simulink model "s0401_DC_motor_Torque_Feedback"  (R2021a)
settings: Solver=VariableStepAuto  StartTime=0.0  StopTime=0.2  RelTol=1e-3
libraries: pid_lib x1
settings Model: Creator=s329046  LastModifiedBy=s329046

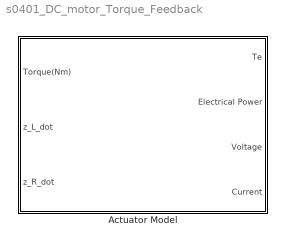
== system s0401_DC_motor_Torque_Feedback ==
  "Actuator Model " : Subsystem

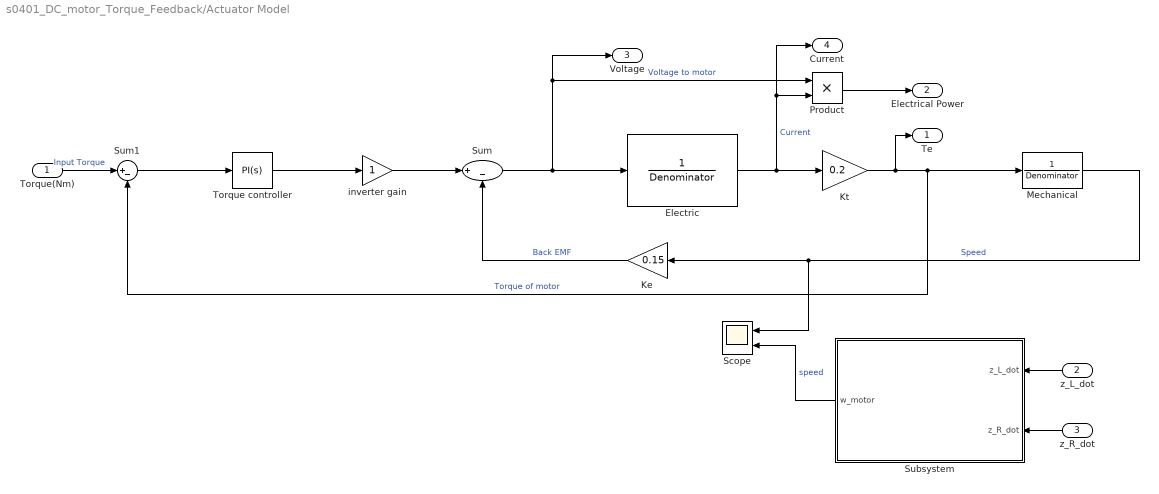
== system s0401_DC_motor_Torque_Feedback/Actuator Model  ==
  Torque(Nm) : Inport
  z_L_dot : Inport  Port=2
  z_R_dot : Inport  Port=3
  "Electric " : TransferFcn  Denominator=Denominator  mask{Denominator=[0.0001 0.8]}
      mask prompts: Denominator "[La Ra]"
      mask TypeOptions Denominator: Denominator
  Ke : Gain  Gain=0.15
  Kt : Gain  Gain=0.2
  Mechanical : TransferFcn  Denominator=Denominator  mask{Denominator=[0.0002 0.042]}
      mask prompts: Denominator "[J B]"
      mask TypeOptions Denominator: Denominator
  Product : Product
  Scope : Scope  NumInputPorts=2
  Subsystem : Subsystem
  Sum : Sum  Inputs=|+-
  Sum1 : Sum  Inputs=|+-
  "Torque controller " : pid_lib/PID Controller  Controller=PI  Form=Parallel  TimeDomain=Continuous-time  UseExternalTs=off  SampleTime=-1  IntegratorMethod=Forward Euler  FilterMethod=Forward Euler  ControllerParametersSource=internal  P=0.59  I=3492  D=0  UseFilter=on  N=100  TunerSelectOption=Transfer Function Based (PID Tuner App)  InitialConditionSource=internal  InitialConditionForIntegrator=0  InitialConditionForFilter=0  DifferentiatorICPrevScaledInput=0  ExternalReset=none  TrackingMode=off  Kt=1  LimitOutput=off  SatLimitsSource=internal  UpperSaturationLimit=inf  LowerSaturationLimit=-inf  LinearizeAsGain=on  AntiWindupMode=none  Kb=1  POutMin=[]  POutMax=[]  IOutMin=[]  IOutMax=[]  DOutMin=[]  DOutMax=[]  NOutMin=[]  NOutMax=[]  SumOutMin=[]  SumOutMax=[]  SaturationOutMin=[]  SaturationOutMax=[]  PParamMin=[]  PParamMax=[]  IParamMin=[]  IParamMax=[]  DParamMin=[]  DParamMax=[]  NParamMin=[]  NParamMax=[]  KbParamMin=[]  KbParamMax=[]  KtParamMin=[]  KtParamMax=[]  KbOutMin=[]  KbOutMax=[]  KtOutMin=[]  KtOutMax=[]  IntegratorOutMin=[]  IntegratorOutMax=[]  FilterOutMin=[]  FilterOutMax=[]  SumI1OutMin=[]  SumI1OutMax=[]  SumI2OutMin=[]  SumI2OutMax=[]  SumI3OutMin=[]  SumI3OutMax=[]  SumI4OutMin=[]  SumI4OutMax=[]  SumDOutMin=[]  SumDOutMax=[]  DifferentiatorOutMin=[]  DifferentiatorOutMax=[]  FilterDiffOutCoefMin=[]  FilterDiffOutCoefMax=[]  ReciprocalOutMin=[]  ReciprocalOutMax=[]  SumDenOutMin=[]  SumDenOutMax=[]  SumNumOutMin=[]  SumNumOutMax=[]  DivideOutMin=[]  DivideOutMax=[]  UdiffTsProdOutMin=[]  UdiffTsProdOutMax=[]  NTsProdOutMin=[]  NTsProdOutMax=[]  UintegralTsProdOutMin=[]  UintegralTsProdOutMax=[]  UngainTsProdOutMin=[]  UngainTsProdOutMax=[]  IntegratorContinuousStateAttributes=''  IntegratorStateMustResolveToSignalObject=off  IntegratorRTWStateStorageClass=Auto  FilterContinuousStateAttributes=''  FilterStateMustResolveToSignalObject=off  FilterRTWStateStorageClass=Auto  ParallelPVariant=InternalParameters  IdealPVariant=Disabled  IVariant=InternalParameters  DVariant=Disabled  IntegratorVariant=Continuous  SatVariant=Disabled  AWVariant=Passthrough  PCopyVariant=Disabled  TRVariant=Disabled  FdbkBlocksVariant=Forward  IdealPFdbkVariant=Disabled  SatFdbkVariant=Disabled  DerivativeFilterVariant=Disabled  NVariant=Disabled  NCopyVariant=Disabled_SignalSpec  FilterICVariant=Disabled  IntegratorICVariant=InternalICs  ExternalResetVariant=Disabled  TRSumVariant=Passthrough  SumFdbkVariant=Disabled  SumVariant=Sum_PI  TsampFilterVariant=InternalTs  TsampNgainVariant=Passthrough  TsampIntegralVariant=Passthrough  ExternalSaturationOutDataTypeStr=Inherit: Same as second input
  inverter gain : Gain
  Te : Outport
  Electrical Power : Outport  Port=2
  Voltage : Outport  Port=3
  Current : Outport  Port=4
  wires:
  inverter gain/1 -> Sum/1
  Ke/1 -> Sum/2  "Back EMF"
  "Electric "/1 -> Current/1, Product/2, Kt/1  "Current"
  "Torque controller "/1 -> inverter gain/1
  Torque(Nm)/1 -> Sum1/1  "Input Torque"
  Sum/1 -> Voltage/1, Product/1, "Electric "/1  "Voltage to motor"
  Kt/1 -> Te/1, Mechanical/1, Sum1/2  "Torque of motor"
  Sum1/1 -> "Torque controller "/1
  Product/1 -> Electrical Power/1
  z_L_dot/1 -> Subsystem/1(z_L_dot)
  z_R_dot/1 -> Subsystem/2(z_R_dot)
  Mechanical/1 -> Scope/1, Ke/1  "Speed"
  Subsystem/1(w_motor) -> Scope/2  "speed"

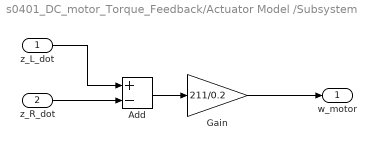
== system s0401_DC_motor_Torque_Feedback/Actuator Model /Subsystem ==
  z_L_dot : Inport
  z_R_dot : Inport  Port=2
  Add : Sum  Inputs=+-
  Gain : Gain  Gain=211/0.2
  w_motor : Outport
  wires:
  z_L_dot/1 -> Add/1
  z_R_dot/1 -> Add/2
  Add/1 -> Gain/1
  Gain/1 -> w_motor/1
